simulink model "VSD_and_Park_transformation_6Phase"  (R2022a)
settings: Solver=FixedStepDiscrete  StartTime=0.0  StopTime=0.2  RelTol=1e-3
undefined symbols (not defined in the file or in its folder): T_100MHz
libraries: simulink x2, hdlsllib x1
settings Model: DataTypeOverride=Off  Creator=Andre Merx  LastModifiedBy=Andre Merx
settings SolverCC: AlgebraicLoopSolver=TrustRegion
settings DataIOCC: LimitDataPoints=on  SaveOutput=off  SaveTime=off
settings OptimizationCC: BlockReduction=off  ConditionallyExecuteInputs=off  DefaultParameterBehavior=Inlined  LifeSpan=inf
settings DebuggingCC: AlgebraicLoopMsg=error  SingleTaskRateTransMsg=error  UnconnectedInputMsg=warning  UnconnectedOutputMsg=warning  UnconnectedLineMsg=warning  AllowSymbolicDim=off  StrictBusMsg=ErrorOnBusTreatedAsVector  SFUnexpectedBacktrackingDiag=warning  SFNoUnconditionalDefaultTransitionDiag=warning  SFExecutionAtInitializationDiag=none  SFMachineParentedDataDiag=warning  ArithmeticOperatorsInVariantConditions=warning
settings HardwareCC: ProdBitPerPointer=32  ProdBitPerSizeT=32  ProdBitPerPtrDiffT=32  ProdLargestAtomicFloat=None  ProdIntDivRoundTo=Undefined  ProdEndianess=Unspecified  ProdWordSize=32  ProdHWDeviceType=ASIC/FPGA->ASIC/FPGA  ProdEqTarget=off
settings SFSimCC: SimUseLocalCustomCode=off  CustomCodeUndefinedFunction=UseInterfaceOnly
settings RTWCC: RTWUseLocalCustomCode=off
settings CodeAppCC: StateflowObjectComments=on
settings GRTTargetCC: TargetLangStandard=C89/C90 (ANSI)
settings ConfigComp: CovScope=ReferencedModels  CovMetricSettings=dw  CovSaveCumulativeToWorkspaceVar=on  CovSaveSingleToWorkspaceVar=on  CovExternalEMLEnable=off  CovSFcnEnable=off

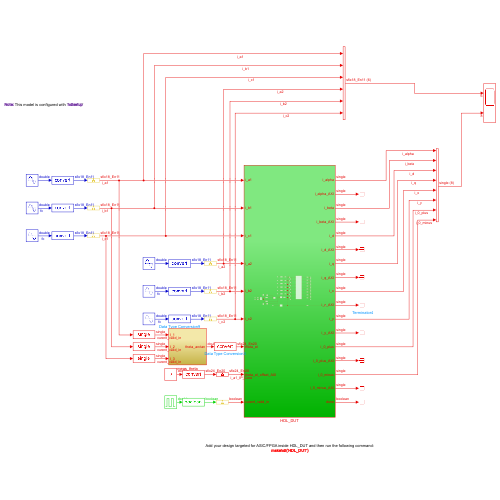
[thumbnail: Simulink's stored preview of the top-level diagram]
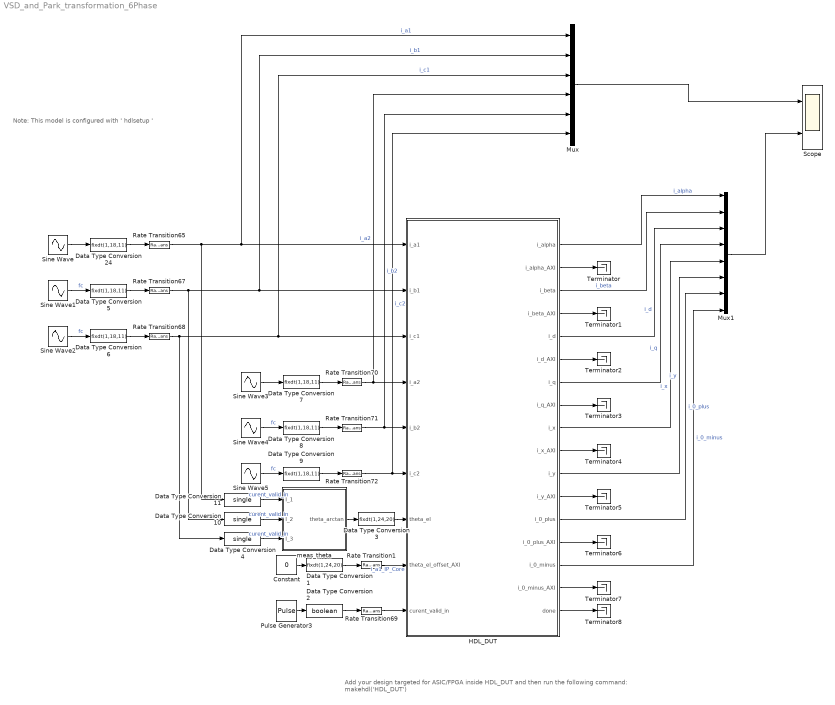
== system VSD_and_Park_transformation_6Phase ==
  note: Note: This model is configured with ' hdlsetup '
  note: Add your design targeted for ASIC/FPGA inside HDL_DUT and then run the following command:
      | makehdl('HDL_DUT')
  Constant : Constant  Value=0  SampleTime=-1
  Data Type Conversion1 : DataTypeConversion  OutDataTypeStr=fixdt(1,24,20)  SaturateOnIntegerOverflow=off  RndMeth=Floor
  Data Type Conversion10 : DataTypeConversion  OutDataTypeStr=single  SaturateOnIntegerOverflow=off  RndMeth=Floor
  Data Type Conversion11 : DataTypeConversion  OutDataTypeStr=single  SaturateOnIntegerOverflow=off  RndMeth=Floor
  Data Type Conversion2 : DataTypeConversion  OutDataTypeStr=boolean  SaturateOnIntegerOverflow=off  RndMeth=Floor
  Data Type Conversion{5..9,24} (6 alike) : DataTypeConversion  OutDataTypeStr=fixdt(1,18,11)  SaturateOnIntegerOverflow=off  RndMeth=Floor
  Data Type Conversion3 : DataTypeConversion  OutDataTypeStr=fixdt(1,24,20)  SaturateOnIntegerOverflow=off  RndMeth=Floor
  Data Type Conversion4 : DataTypeConversion  OutDataTypeStr=single  SaturateOnIntegerOverflow=off  RndMeth=Floor
  HDL_DUT : Subsystem
  Mux : Mux  Inputs=6
  Mux1 : Mux  Inputs=8
  Pulse Generator3 : DiscretePulseGenerator  PulseType=Time based  Period=1/100000  PulseWidth=5
  Rate Transition{1,65,67..72} (8 alike) : RateTransition  OutPortSampleTime=1.0000e-08
  Scope : Scope  NumInputPorts=2
  Sine Wave : Sin  Frequency=100  SampleTime=1/100000
  Sine Wave1 : Sin  Frequency=100  Phase=(4/3)*pi  SampleTime=1/100000
  Sine Wave2 : Sin  Frequency=100  Phase=(2/3)*pi  SampleTime=1/100000
  Sine Wave3 : Sin  Amplitude=0.5  Frequency=100  Phase=-pi/6  SampleTime=1/100000
  Sine Wave4 : Sin  Amplitude=0.5  Frequency=100  Phase=(7/6)*pi  SampleTime=1/100000
  Sine Wave5 : Sin  Amplitude=0.5  Frequency=100  Phase=(1/2)*pi  SampleTime=1/100000
  Terminator{,1..8} (9 alike) : Terminator
  meas_theta : Subsystem
  wires:
  Sine Wave/1 -> Data Type Conversion24/1
  Sine Wave1/1 -> Data Type Conversion5/1  "fc"
  Data Type Conversion6/1 -> Rate Transition68/1
  Sine Wave2/1 -> Data Type Conversion6/1  "fc"
  Data Type Conversion5/1 -> Rate Transition67/1
  Data Type Conversion24/1 -> Rate Transition65/1
  Rate Transition65/1 -> Mux/1, HDL_DUT/1(i_a1), Data Type Conversion11/1  "i_a1"
  Rate Transition67/1 -> Mux/2, HDL_DUT/2(i_b1), Data Type Conversion10/1  "i_b1"
  Rate Transition68/1 -> Mux/3, HDL_DUT/3(i_c1), Data Type Conversion4/1  "i_c1"
  Sine Wave5/1 -> Data Type Conversion9/1  "fc"
  Data Type Conversion9/1 -> Rate Transition72/1
  Sine Wave4/1 -> Data Type Conversion8/1  "fc"
  Sine Wave3/1 -> Data Type Conversion7/1
  Data Type Conversion7/1 -> Rate Transition70/1
  Data Type Conversion8/1 -> Rate Transition71/1
  Rate Transition70/1 -> Mux/4, HDL_DUT/4(i_a2)  "i_a2"
  Rate Transition71/1 -> Mux/5, HDL_DUT/5(i_b2)  "i_b2"
  Rate Transition72/1 -> Mux/6, HDL_DUT/6(i_c2)  "i_c2"
  meas_theta/1(theta_arctan) -> Data Type Conversion3/1
  Constant/1 -> Data Type Conversion1/1
  Data Type Conversion1/1 -> Rate Transition1/1
  Rate Transition1/1 -> HDL_DUT/8(theta_el_offset_AXI)  "i_a1_IP_Core"
  Pulse Generator3/1 -> Data Type Conversion2/1
  Rate Transition69/1 -> HDL_DUT/9(curent_valid_in)
  Data Type Conversion2/1 -> Rate Transition69/1
  HDL_DUT/2(i_alpha_AXI) -> Terminator/1
  HDL_DUT/4(i_beta_AXI) -> Terminator1/1
  HDL_DUT/6(i_d_AXI) -> Terminator2/1
  HDL_DUT/8(i_q_AXI) -> Terminator3/1
  HDL_DUT/10(i_x_AXI) -> Terminator4/1
  HDL_DUT/12(i_y_AXI) -> Terminator5/1
  HDL_DUT/14(i_0_plus_AXI) -> Terminator6/1
  HDL_DUT/16(i_0_minus_AXI) -> Terminator7/1
  HDL_DUT/17(done) -> Terminator8/1
  Mux/1 -> Scope/1
  HDL_DUT/1(i_alpha) -> Mux1/1  "i_alpha"
  HDL_DUT/3(i_beta) -> Mux1/2  "i_beta"
  HDL_DUT/5(i_d) -> Mux1/3  "i_d"
  HDL_DUT/7(i_q) -> Mux1/4  "i_q"
  HDL_DUT/9(i_x) -> Mux1/5  "i_x"
  HDL_DUT/11(i_y) -> Mux1/6  "i_y"
  HDL_DUT/13(i_0_plus) -> Mux1/7  "i_0_plus"
  HDL_DUT/15(i_0_minus) -> Mux1/8  "i_0_minus"
  Mux1/1 -> Scope/2
  Data Type Conversion3/1 -> HDL_DUT/7(theta_el)
  Data Type Conversion4/1 -> meas_theta/3(I_3)  "curent_valid_in"
  Data Type Conversion10/1 -> meas_theta/2(I_2)  "curent_valid_in"
  Data Type Conversion11/1 -> meas_theta/1(I_1)  "curent_valid_in"

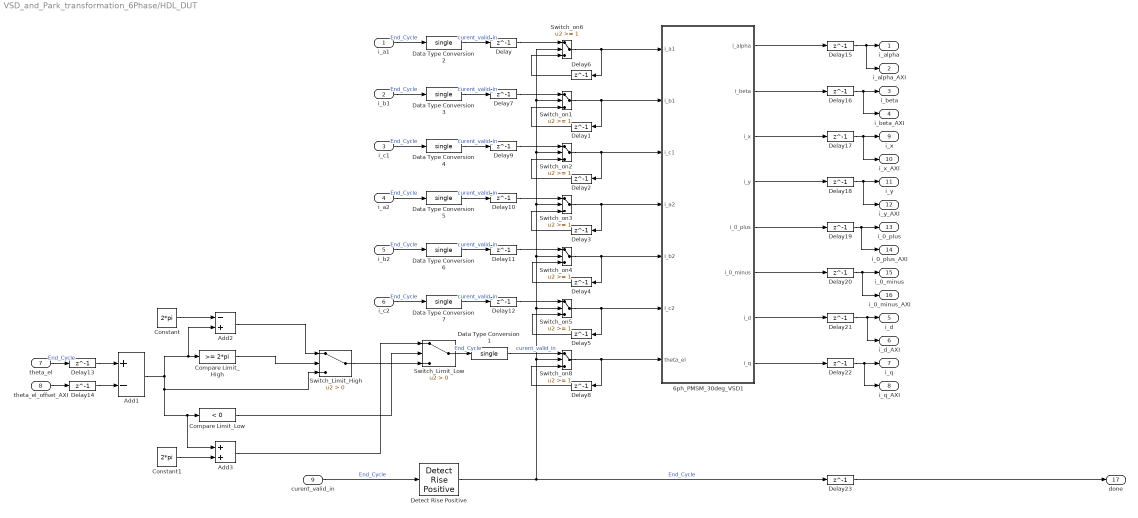
== system VSD_and_Park_transformation_6Phase/HDL_DUT ==
  i_a1 : Inport
  i_b1 : Inport  Port=2
  i_c1 : Inport  Port=3
  i_a2 : Inport  Port=4
  i_b2 : Inport  Port=5
  i_c2 : Inport  Port=6
  theta_el : Inport  Port=7
  theta_el_offset_AXI : Inport  Port=8
  curent_valid_in : Inport  Port=9
  6ph_PMSM_30deg_VSD1 : MATLAB Function  TreatAsAtomicUnit=on  SystemSampleTime=T_100MHz
  Add1 : Sum  Inputs=+-  OutDataTypeStr=Inherit: Same as accumulator
  Add2 : Sum  Inputs=-+  OutDataTypeStr=Inherit: Same as first input
  Add3 : Sum  OutDataTypeStr=Inherit: Same as first input
  Compare Limit_High : simulink/Logic and Bit Operations/Compare To Constant  relop=>=  const=2*pi  OutDataTypeStr=boolean
  Compare Limit_Low : simulink/Logic and Bit Operations/Compare To Constant  relop=<  const=0  OutDataTypeStr=boolean
  Constant : Constant  Value=2*pi  OutDataTypeStr=single  SampleTime=T_100MHz
  Constant1 : Constant  Value=2*pi  OutDataTypeStr=single  SampleTime=T_100MHz
  Data Type Conversion{1..7} (7 alike) : DataTypeConversion  OutDataTypeStr=single  SaturateOnIntegerOverflow=off  RndMeth=Floor
  Delay{,1..23} (24 alike) : Delay  DelayLength=1
  Detect Rise Positive : hdlsllib/Logic and Bit Operations/Detect Rise Positive  vinit=0  OutDataTypeStr=boolean
      settings: SourceProductBaseCode=SL
  Switch_Limit_High : Switch  Criteria=u2 > Threshold  OutDataTypeStr=single  SaturateOnIntegerOverflow=off  InputSameDT=off
  Switch_Limit_Low : Switch  Criteria=u2 > Threshold  OutDataTypeStr=single  SaturateOnIntegerOverflow=off  InputSameDT=off
  Switch_on{1..6,8} (7 alike) : Switch  Threshold=1  OutDataTypeStr=single  RndMeth=Simplest  SaturateOnIntegerOverflow=off  InputSameDT=off
  i_alpha : Outport
  i_alpha_AXI : Outport  Port=2
  i_beta : Outport  Port=3
  i_beta_AXI : Outport  Port=4
  i_d : Outport  Port=5
  i_d_AXI : Outport  Port=6
  i_q : Outport  Port=7
  i_q_AXI : Outport  Port=8
  i_x : Outport  Port=9
  i_x_AXI : Outport  Port=10
  i_y : Outport  Port=11
  i_y_AXI : Outport  Port=12
  i_0_plus : Outport  Port=13
  i_0_plus_AXI : Outport  Port=14
  i_0_minus : Outport  Port=15
  i_0_minus_AXI : Outport  Port=16
  done : Outport  Port=17
  wires:
  Switch_Limit_Low/1 -> Data Type Conversion1/1  "End_Cycle"
  theta_el_offset_AXI/1 -> Delay14/1
  i_c2/1 -> Data Type Conversion7/1  "End_Cycle"
  Switch_on8/1 -> 6ph_PMSM_30deg_VSD1/7(theta_el), Delay8/1
  Delay8/1 -> Switch_on8/3
  Detect Rise Positive/1 -> Switch_on6/2, Switch_on1/2, Switch_on2/2, Switch_on3/2, Switch_on4/2, Switch_on5/2, Switch_on8/2, Delay23/1  "End_Cycle"
  Delay4/1 -> Switch_on4/3
  Switch_on2/1 -> Delay2/1, 6ph_PMSM_30deg_VSD1/3(i_c1)
  6ph_PMSM_30deg_VSD1/8(i_q) -> Delay22/1
  Delay1/1 -> Switch_on1/3
  6ph_PMSM_30deg_VSD1/5(i_0_plus) -> Delay19/1
  Switch_on1/1 -> Delay1/1, 6ph_PMSM_30deg_VSD1/2(i_b1)
  Switch_on6/1 -> Delay6/1, 6ph_PMSM_30deg_VSD1/1(i_a1)
  Switch_on4/1 -> Delay4/1, 6ph_PMSM_30deg_VSD1/5(i_b2)
  6ph_PMSM_30deg_VSD1/3(i_x) -> Delay17/1
  curent_valid_in/1 -> Detect Rise Positive/1  "End_Cycle"
  6ph_PMSM_30deg_VSD1/7(i_d) -> Delay21/1
  6ph_PMSM_30deg_VSD1/1(i_alpha) -> Delay15/1
  6ph_PMSM_30deg_VSD1/6(i_0_minus) -> Delay20/1
  Switch_Limit_High/1 -> Switch_Limit_Low/3
  Switch_on3/1 -> Delay3/1, 6ph_PMSM_30deg_VSD1/4(i_a2)
  6ph_PMSM_30deg_VSD1/4(i_y) -> Delay18/1
  Add1/1 -> Switch_Limit_High/3, Add3/1, Compare Limit_Low/1, Add2/2, Compare Limit_High/1
  Delay6/1 -> Switch_on6/3
  Constant/1 -> Add2/1
  Data Type Conversion1/1 -> Switch_on8/1  "curent_valid_in"
  Compare Limit_High/1 -> Switch_Limit_High/2
  Compare Limit_Low/1 -> Switch_Limit_Low/2
  Delay2/1 -> Switch_on2/3
  Constant1/1 -> Add3/2
  theta_el/1 -> Delay13/1  "End_Cycle"
  Delay3/1 -> Switch_on3/3
  i_a1/1 -> Data Type Conversion2/1  "End_Cycle"
  i_b2/1 -> Data Type Conversion6/1  "End_Cycle"
  Add2/1 -> Switch_Limit_High/1
  i_a2/1 -> Data Type Conversion5/1  "End_Cycle"
  i_b1/1 -> Data Type Conversion3/1  "End_Cycle"
  Delay5/1 -> Switch_on5/3
  Add3/1 -> Switch_Limit_Low/1
  i_c1/1 -> Data Type Conversion4/1  "End_Cycle"
  6ph_PMSM_30deg_VSD1/2(i_beta) -> Delay16/1
  Switch_on5/1 -> Delay5/1, 6ph_PMSM_30deg_VSD1/6(i_c2)
  Delay/1 -> Switch_on6/1
  Delay7/1 -> Switch_on1/1
  Delay9/1 -> Switch_on2/1
  Delay10/1 -> Switch_on3/1
  Delay11/1 -> Switch_on4/1
  Delay12/1 -> Switch_on5/1
  Delay13/1 -> Add1/1
  Delay14/1 -> Add1/2
  Delay15/1 -> i_alpha_AXI/1, i_alpha/1
  Delay16/1 -> i_beta_AXI/1, i_beta/1
  Delay17/1 -> i_x_AXI/1, i_x/1
  Delay18/1 -> i_y_AXI/1, i_y/1
  Delay19/1 -> i_0_plus_AXI/1, i_0_plus/1
  Delay20/1 -> i_0_minus_AXI/1, i_0_minus/1
  Delay21/1 -> i_d_AXI/1, i_d/1
  Delay22/1 -> i_q_AXI/1, i_q/1
  Delay23/1 -> done/1
  Data Type Conversion2/1 -> Delay/1  "curent_valid_in"
  Data Type Conversion3/1 -> Delay7/1  "curent_valid_in"
  Data Type Conversion4/1 -> Delay9/1  "curent_valid_in"
  Data Type Conversion5/1 -> Delay10/1  "curent_valid_in"
  Data Type Conversion6/1 -> Delay11/1  "curent_valid_in"
  Data Type Conversion7/1 -> Delay12/1  "curent_valid_in"

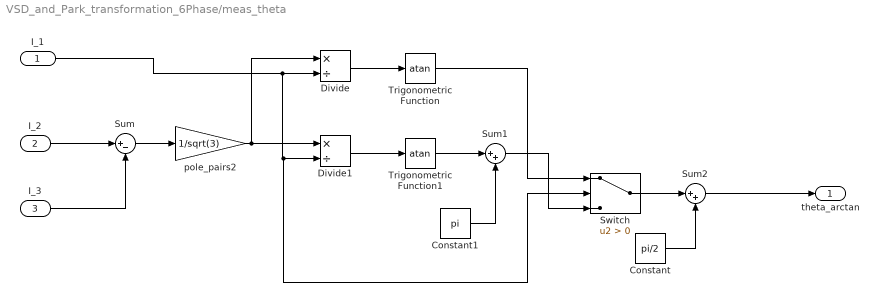
== system VSD_and_Park_transformation_6Phase/meas_theta ==
  I_1 : Inport
  I_2 : Inport  Port=2
  I_3 : Inport  Port=3
  Constant : Constant  Value=pi/2
  Constant1 : Constant  Value=pi
  Divide : Product  Inputs=*/
  Divide1 : Product  Inputs=*/
  Sum : Sum  Inputs=|+-
  Sum1 : Sum  Inputs=|++
  Sum2 : Sum  Inputs=|++
  Switch : Switch  Criteria=u2 > Threshold  SaturateOnIntegerOverflow=off  InputSameDT=off
  Trigonometric Function : Trigonometry  Operator=atan
  Trigonometric Function1 : Trigonometry  Operator=atan
  pole_pairs2 : Gain  Gain=1/sqrt(3)
  theta_arctan : Outport  VectorParamsAs1DForOutWhenUnconnected=off
  wires:
  Divide/1 -> Trigonometric Function/1
  Divide1/1 -> Trigonometric Function1/1
  Trigonometric Function1/1 -> Sum1/1
  pole_pairs2/1 -> Divide/1, Divide1/1
  Sum/1 -> pole_pairs2/1
  I_3/1 -> Sum/2
  I_2/1 -> Sum/1
  I_1/1 -> Switch/2, Divide1/2, Divide/2
  Sum1/1 -> Switch/3
  Trigonometric Function/1 -> Switch/1
  Switch/1 -> Sum2/1
  Constant/1 -> Sum2/2
  Constant1/1 -> Sum1/2
  Sum2/1 -> theta_arctan/1

== matlab function VSD_and_Park_transformation_6Phase/HDL_DUT/6ph_PMSM_30deg_VSD1 ==
  data: i_a1 input; i_alpha output; i_b1 input; i_c1 input; i_a2 input; i_b2 input; i_c2 input; theta_el input; i_beta output; i_x output; i_y output; i_0_plus output; i_0_minus output; i_d output; i_q output
function [i_alpha,i_beta,i_x,i_y,i_0_plus,i_0_minus,i_d,i_q] = VSD_and_Park_transformation(i_a1,i_b1,i_c1,i_a2,i_b2,i_c2,theta_el)

    % VSD-Transformation
    A =[0 0 0 0 0 0]';

    A =    (1/3)*[1    -0.5        -0.5        sqrt(3)/2   -sqrt(3)/2  0 ;
                  0    sqrt(3)/2   -sqrt(3)/2  0.5         0.5         -1;
                  1    -0.5        -0.5        -sqrt(3)/2  sqrt(3)/2   0 ;
                  0    -sqrt(3)/2  sqrt(3)/2   0.5         0.5         -1;
                  1    1           1           0           0           0 ;
                  0    0           0           1           1           1] * [i_a1 i_b1 i_c1 i_a2 i_b2 i_c2]';

    i_alpha = A(1);
    i_beta = A(2);
    i_x = A(3);
    i_y = A(4);
    i_0_plus = A(5);
    i_0_minus = A(6);

    % Park-Transformation

    B = [0 0]';

     B = [cos(theta_el)       sin(theta_el);
         -sin(theta_el)       cos(theta_el)] * [i_alpha i_beta]';

    i_d = B(1);
    i_q = B(2);

end
